simulink model "Model_plane2_new_Old_vers"  (R2021b)
settings: Solver=FixedStepAuto  StartTime=0  StopTime=3000  FixedStep=1  RelTol=1e-3
model workspace (MAT data in the model file):
  Alfa = [-2 4 10 16]
  Alfa_RUD = 0.55
  Alfa_table = [-4 0 5 10 20]
  Alfa_y = [-4 6 8 9 10 12 14]
  Cxa_table = [0.03434 0.02598 0.04151 0.122 0.502 0.0358 0.0252 0.0505 0.1649 0.538 0.04274 0.0262 ... (15 elements, 5x3)]
  Cy_DB = [0.01242 0.01286 0.01457]
  Cy_fi = [0.00623 0.00643 0.00626]
  Cya = [-0.276 0.859 1.085 1.2 1.296 1.45 1.461 -0.33 0.991 1.211 1.275 1.29 ... (21 elements, 7x3)]
  Del_B = -5
  H = [339 3256 4060 8000 12000]
  H_table = [0 2000 4000 6000 8000 10000]
  I = [1000 1000 4500000]
  K_dH = -0.3
  K_p = 0.3
  K_roll = 1
  K_w = 1.5
  K_wx = 1
  K_wy = 1
  Ki_H = 1e-05
  Ki_P = 1
  Ki_V = 0.009
  Ki_n = 1
  Kp_H = 0.03
  Kp_P = 1
  Kp_V = 0.9
  Kp_n = 1
  M_C = [0.4 0.6 0.82]
  M_mz = [0.2 0.4 0.6 0.8]
  M_mz2 = [0.4 0.7 0.85]
  M_table = [0.4 0.7 0.82]
  M_y = [0.4 0.7 0.82]
  P = [70000 56000 44800 35840 28672]
  Psi0 = 0
  Skr = 131
  Teta0 = 0
  V0 = 135
  a_table = [340.3 339.5 338.8 338 337.2 336.4]
  ba = 3.466
  fi = 0
  fi_P = 2
  g = 9.81
  lz = 4500000
  mla = 60000
  mz_DB = [-0.035 -0.0358 -0.037 -0.0377]
  mz_alfa = [-0.0282 -0.0282 -0.0289 -0.0404]
  mz_alfa2 = [-8.163  -8.762  -9.714; -8.163  -8.762  -9.583; -7.975  -7.991  -7.868; -6.514  -6.413  -6.732]
  mz_fi = [-0.0695 -0.0714 -0.0739 -0.0832]
  mz_omz = [-23.768  -25.3  -28.284; -23.768  -25.3  -27.903; -23.222  -22.6  -23.32; -18.967  -18.52  -19.601]
  n_dvig = 2
  out : Simulink.SimulationOutput (value not decoded)
  pitch = 1
  pitch0 = 0
  q_table = [1.225 1.0065 0.8194 0.6601 0.5258 0.4135]
  roll0 = 0
  wx0 = 0
  wy0 = 0
  wz0 = 0
  x0 = 0
  xy = [240000 6200]
  y0 = 5000
  yaw0 = 0
  z0 = 0
libraries: simulink x10
(part 2 of 2)

== matlab function Model_plane2_new_Old_vers/Динамика самолёта/Вектор внешних сил/MATLAB Function ==
  data: mla input; l input; W output; g input; k input
function W = fcn(mla,l,g,k)
W=[-k*mla*g;-l*mla*g;0];

== matlab function Model_plane2_new_Old_vers/Динамика самолёта/Вектор проекций аэродинамических сил/MATLAB Function ==
  data: A input; Fk output; P input; W input; Teta input; Psi input; Alfa input; Beta input; roll_a input; yaw input; pitch input; roll input
function Fk = fcn(A,P,W,Teta,Psi,Alfa,Beta,roll_a,yaw,pitch,roll)

yaw_a=Psi;
pitch_a=Teta;


D_g_k = [cos(Psi)*cos(Teta), sin(Teta), -sin(Psi)*cos(Teta);
        -cos(Psi)*sin(Teta), cos(Teta), sin(Psi)*sin(Teta);
        sin(Psi), 0, cos(Psi)];

D_gv = [cos(yaw_a)*cos(pitch_a), sin(pitch_a), -sin(yaw_a)*cos(pitch_a);
        -cos(yaw_a)*sin(pitch_a)*cos(roll_a) + sin(yaw_a)*sin(roll_a), cos(pitch_a)*cos(roll_a), cos(yaw_a)*sin(roll_a) + sin(yaw_a)*sin(pitch_a)*cos(roll_a);
        cos(yaw_a)*sin(pitch_a)*sin(roll_a) + sin(yaw_a)*cos(roll_a), -cos(pitch_a)*sin(roll_a), cos(yaw_a)*cos(roll_a) - sin(yaw_a)*sin(pitch_a)*sin(roll_a)];
 
D_g_cv=[cos(yaw)*cos(pitch), sin(pitch), -sin(yaw)*cos(pitch);
    sin(yaw)*sin(roll)-cos(yaw)*sin(pitch)*cos(roll), cos(pitch)*cos(roll), cos(yaw)*sin(roll)+sin(yaw)*sin(pitch)*cos(roll);
    sin(yaw)*cos(roll)+cos(yaw)*sin(pitch)*sin(roll), -cos(pitch)*sin(roll), cos(yaw)*cos(roll)-sin(yaw)*sin(pitch)*sin(roll)];

D_cv_a = [cos(Alfa)*cos(Beta), -sin(Alfa)*cos(Beta), sin(Beta);
        sin(Alfa), cos(Alfa), 0;
        -cos(Alfa)*sin(Beta), sin(Alfa)*sin(Beta), cos(Beta)];

Fk = D_g_k * (D_g_cv' * (D_cv_a' * A + P) + W);

== matlab function Model_plane2_new_Old_vers/Динамика самолёта/Блок расчёта параметров стандартной атмосферы/MATLAB Function ==
  data: ro input; a input; q output; V input; M output
function [q, M] = fcn(ro, a, V)

q=(ro*V^2)/2;
M=V/a;

== matlab function Model_plane2_new_Old_vers/Динамика самолёта/Расчёт вектора мометнов Mx,My,Mz/Расчёт M_x (момент крена)/MATLAB Function ==
  data: u input; M_x output
function M_x = fcn(u)
c=0;

M_x = c*u;

== matlab function Model_plane2_new_Old_vers/Динамика самолёта/Вектор тяги двигателя/Проекции аэродинамических сил ==
  data: Px output; fi_p input; P input; alfa_Rud input; n_dvig input; Py output
function [Px, Py] = fcn(fi_p,P,alfa_Rud,n_dvig)

Px=cos(fi_p)*(n_dvig*alfa_Rud*P);
Py=sin(fi_p)*(n_dvig*alfa_Rud*P);

== matlab function Model_plane2_new_Old_vers/Динамика самолёта/Расчёт вектора мометнов Mx,My,Mz/Вектор моментов ==
  data: M_x input; M output; M_y input; M_z input
function M = fcn(M_x, M_y, M_z)

M=[M_x; M_y; M_z];
